simulink model "sopc_edge_detector"  (Simulink 6.3)
settings: Solver=FixedStepDiscrete  SolverMode=SingleTasking  StartTime=0.0  StopTime=307201.0  RelTol=1e-3
InitFcn:
  | ed_in_script
  | %% DSPBuilder Start
  | alt_dspbuilder_update_model(bdroot)
  | %% DSPBuilder End
StopFcn:
  | ed_out_script
libraries: allblocks_alteradspbuilder2 x63
settings Model: Creator=sichou  LastModifiedBy=LKONG
settings DataIOCC: SignalLoggingName=sigsOut
settings OptimizationCC: InlineInvariantSignals=on
settings DebuggingCC: AlgebraicLoopMsg=none  ArtificialAlgebraicLoopMsg=none  CheckExecutionContextPreStartOutputMsg=on  CheckExecutionContextRuntimeOutputMsg=on  SolverPrmCheckMsg=none
settings HardwareCC: TargetHWDeviceType=32-bit Generic  ProdEqTarget=off

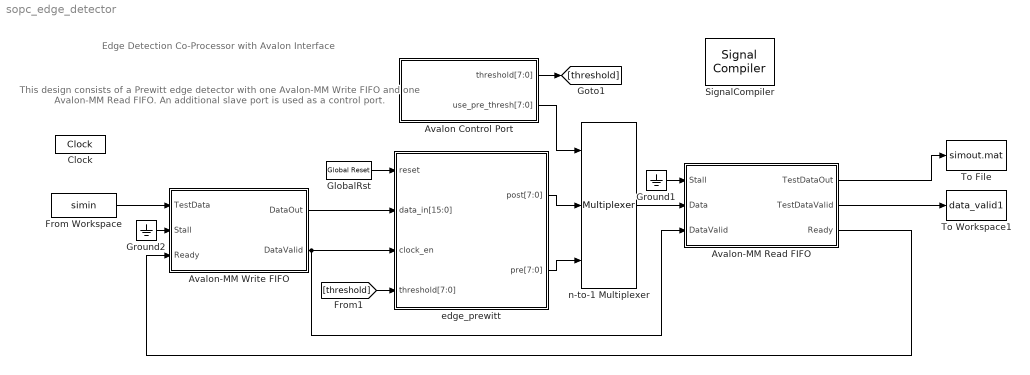
== system sopc_edge_detector ==
  note: Edge Detection Co-Processor
      | with Avalon Interface
  note: This design consists of a Prewitt edge detector with one Avalon-MM
      | Write FIFO and one Avalon-MM Read FIFO.  An additional slave port
      | is used as a control port.
  Avalon Control Port : Subsystem
      mask Type: SubSystem AlteraBlockSet
  Avalon-MM Read FIFO : Subsystem  mask(Avalon-MM Read FIFO AlteraBlockSet){sgn=Unsigned Integer, bwl=8, bwr=0, depth=16, burst=8}
      mask prompts: sgn "Data Type"; bwl "[number of bits].[]"; bwr "[].[number of bits]"; depth "FIFO Depth"; burst "Max Burst"
      mask help:
      | Avalon-MM Read FIFO
      |
      | Implements a FIFO with Avalon-MM connectivity. Accessed by other Avalon-MM peripherals to obtain datawhen connected in SOPC Builder.
      |
      | Inputs:
      | Stall - Connect to Simulink blocks.
      | 	Used to simulate stall conditions of the Avalon-MM bus.
      | Data - Connect to DSP Builder blocks.
      | 	Used to collect outgoing data from the user design.
      | DataValid - Connect to DSP Builder blocks.
      | 	Should be asserted whenever the signal on the Data port corresponds to real data.
      |
      | Outputs:
      | TestDataOut - Connect to Simulink blocks.
      | 	Corresponds to the data received over the Avalon-MM bus.
      | TestDataValid - Connect to Simulink blocks.
      | 	Asserted whenever TestDataOut corresponds to real data.
      | Ready	- Connect to DSP Builder blocks.
      | 	Used to indicate that the block is ready to receive data.
      mask init:
      | alt_dspbuilder_internal_AvalonFIFO_Init(gcb,1,1, bwl,bwr,depth,burst);
      settings: CopyFcn=set_param(gcbh,'LinkStatus','none');
      mask Help: helpview(fullfile(alt_dspbuilder_get_quartus_rootdir, 'dsp_builder', 'docs', 'AvalonReadFIFO.html'))
      mask StyleString: popup(Signed Integer|Signed Fractional|Unsigned Integer),edit,edit,edit,edit
      mask CallbackString: alt_dspbuilder_internal_AvalonFIFO_Init(gcb,1,0);||||
  Avalon-MM Write FIFO : Subsystem  mask(Avalon-MM Write FIFO AlteraBlockSet){sgn=Unsigned Integer, bwl=8, bwr=0, depth=16, burst=8}
      mask prompts: sgn "Data Type"; bwl "[number of bits].[]"; bwr "[].[number of bits]"; depth "FIFO Depth"; burst "Maximum Burst Size"
      mask help:
      | Avalon-MM Write FIFO
      |
      | Implements a FIFO with Avalon-MM connectivity. Used to receive data from other Avalon-MM peripheralswhen connected in SOPC Builder.
      |
      | Inputs:
      | TestData - Connect to Simulink blocks.
      | 	Used to provide simulation data to the Avalon-MM Write FIFO.
      | Stall - Connect to Simulink blocks.
      | 	Used to simulate stall conditions of the Avalon-MM bus.
      | Ready - Connect to DSP Builder blocks.
      | 	Used to indicate that the downstream hardware is ready for data.
      |
      | Outputs:
      | DataOut - Connect to DSP Builder blocks.
      | 	Corresponds to the oldest unsent data sample received on the TestData port.
      | DataValid - Connect to DSP Builder blocks.
      | 	Asserted whenever DataOut corresponds to real data.
      mask init:
      | alt_dspbuilder_internal_AvalonFIFO_Init(gcb,0,1, bwl,bwr,depth,burst);
      settings: CopyFcn=set_param(gcbh,'LinkStatus','none');
      mask Help: helpview(fullfile(alt_dspbuilder_get_quartus_rootdir, 'dsp_builder', 'docs', 'AvalonWriteFifo.html'))
      mask StyleString: popup(Signed Integer|Signed Fractional|Unsigned Integer),edit,edit,edit,edit
      mask CallbackString: alt_dspbuilder_internal_AvalonFIFO_Init(gcb,0,0);||||
  Clock : allblocks_alteradspbuilder2/Clock  ClockPeriod=100  ClockPeriodUnit=ns  SampleTime=1  SimulationStartCycle=5  PhaseOffset=0  Reset=aclr  ResetType=Active Low  Export=off
  From Workspace : FromWorkspace  VariableName=simin  SampleTime=1
  GlobalRst : allblocks_alteradspbuilder2/Global Reset  SpecifyClock=off
  Ground1 : Ground
  Ground2 : Ground
  SignalCompiler : allblocks_alteradspbuilder2/Signal Compiler  DeviceFamily=Stratix III  DeviceName=AUTO  EnableSignalTap=off  SignalTapDepth=128  UseBoardBlock=off  StpUseDefaultClock=on  StpClock=Clock
  To File : ToFile  Filename=simout.mat  MatrixName=simout
  To Workspace1 : ToWorkspace  VariableName=data_valid1  SampleTime=-1  SaveFormat=Array
  edge_prewitt : Subsystem
      mask Type: SubSystem AlteraBlockSet
  n-to-1 Multiplexer : allblocks_alteradspbuilder2/Multiplexer  numInputs=2  pipeline=0  oneHot=off  use_ena=off  use_aclr=off
  wires:
  Avalon-MM Write FIFO/1(DataOut) -> edge_prewitt/2(data_in[15:0])
  Avalon-MM Write FIFO/2(DataValid) -> edge_prewitt/3(clock_en), Avalon-MM Read FIFO/3(DataValid)
  Avalon-MM Read FIFO/3(Ready) -> Avalon-MM Write FIFO/3(Ready)
  GlobalRst/1 -> edge_prewitt/1(reset)
  Ground2/1 -> Avalon-MM Write FIFO/2(Stall)
  From Workspace/1 -> Avalon-MM Write FIFO/1(TestData)
  edge_prewitt/1(post[7:0]) -> n-to-1 Multiplexer/2
  Ground1/1 -> Avalon-MM Read FIFO/1(Stall)
  Avalon-MM Read FIFO/1(TestDataOut) -> To File/1
  Avalon-MM Read FIFO/2(TestDataValid) -> To Workspace1/1
  Avalon Control Port/2(use_pre_thresh[7:0]) -> n-to-1 Multiplexer/1
  n-to-1 Multiplexer/1 -> Avalon-MM Read FIFO/2(Data)
  edge_prewitt/2(pre[7:0]) -> n-to-1 Multiplexer/3
  Avalon Control Port/1(threshold[7:0]) -> [threshold]
  [threshold] -> edge_prewitt/4(threshold[7:0])

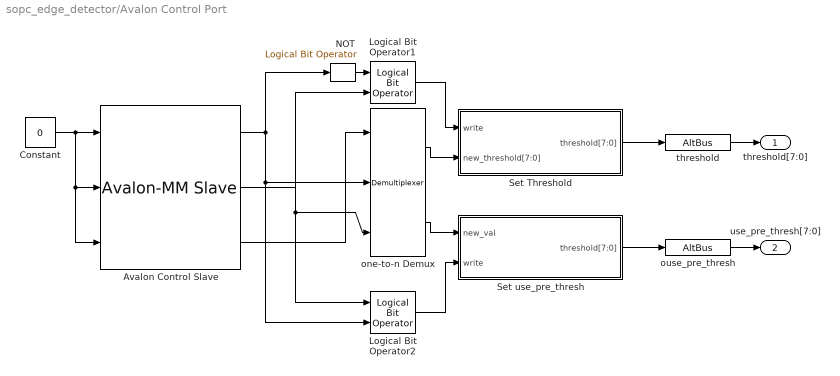
== system sopc_edge_detector/Avalon Control Port ==
  Avalon Control Slave : allblocks_alteradspbuilder2/Avalon-MM Slave  iofile=d:\wsTrunk\workspace\Documentation\DesignExamples\Tutorials\SOPCBuilder\AvalonFIFO\tb_sopc_edge_detector\sopc_edge_detector_Avalon+Control+Port_Avalon+Control+Slave_address.salt,d:\wsTrunk\workspace\Documentation\DesignExamples\Tutorials\SOPCBuilder\AvalonFIFO\tb_sopc_edge_detector\sopc_edge_detector_Avalon+Control+Port_Avalon+Control+Slave_write.salt,d:\wsTrunk\workspace\Documentation\DesignExamples\Tutorials\SOPCBuilder\AvalonFIFO\tb_sopc_edge_detector\sopc_edge_detector_Avalon+Control+Port_Avalon+Control+Slave_writedata.salt,  SpecifyClock=off  clock=clock  addrWidth=1  addrAlignment=Dynamic  addrType=Write  BusType=Unsigned Integer  bwl=8  bwr=0  byteEnable=off  flowCtrl=off  pipeline=off  waitStateFormat=Fixed  readWaitStateCycles=1  writeWaitStateCycles=0  readLatencyFormat=Fixed  readLatencyCycles=0  burst=off  maxBurst=8  irq=off  receiveBeginTransfer=off  useChipSelect=off  PORTTYPE=Output
  Constant : Constant  Value=0
  Logical Bit Operator1 : allblocks_alteradspbuilder2/Logical Bit Operator  LogicalOperator=AND  user_inputs=2
  Logical Bit Operator2 : allblocks_alteradspbuilder2/Logical Bit Operator  LogicalOperator=AND  user_inputs=2
  NOT : allblocks_alteradspbuilder2/Logical Bit Operator  LogicalOperator=NOT  user_inputs=2
  Set Threshold : Subsystem
      mask Type: SubSystem AlteraBlockSet
  Set use_pre_thresh : Subsystem
      mask Type: SubSystem AlteraBlockSet
  one-to-n Demux : allblocks_alteradspbuilder2/Demultiplexer  numOutputs=2  use_ena=on  use_sclr=off
  ouse_pre_thresh : allblocks_alteradspbuilder2/AltBus  BusType=Signed Integer  bwl=8  bwr=0  saturate=off
  threshold : allblocks_alteradspbuilder2/AltBus  BusType=Signed Integer  bwl=8  bwr=0  saturate=off
  threshold[7:0] : Outport
  use_pre_thresh[7:0] : Outport  Port=2
  wires:
  ouse_pre_thresh/1 -> use_pre_thresh[7:0]/1
  Avalon Control Slave/1 -> one-to-n Demux/2, Logical Bit Operator2/2, NOT/1
  Avalon Control Slave/2 -> Logical Bit Operator1/2, one-to-n Demux/3, Logical Bit Operator2/1
  Avalon Control Slave/3 -> one-to-n Demux/1
  one-to-n Demux/1 -> Set Threshold/2(new_threshold[7:0])
  Set use_pre_thresh/1(threshold[7:0]) -> ouse_pre_thresh/1
  NOT/1 -> Logical Bit Operator1/1
  Logical Bit Operator1/1 -> Set Threshold/1(write)
  Logical Bit Operator2/1 -> Set use_pre_thresh/2(write)
  one-to-n Demux/2 -> Set use_pre_thresh/1(new_val)
  threshold/1 -> threshold[7:0]/1
  Set Threshold/1(threshold[7:0]) -> threshold/1
  Constant/1 -> Avalon Control Slave/1, Avalon Control Slave/2, Avalon Control Slave/3

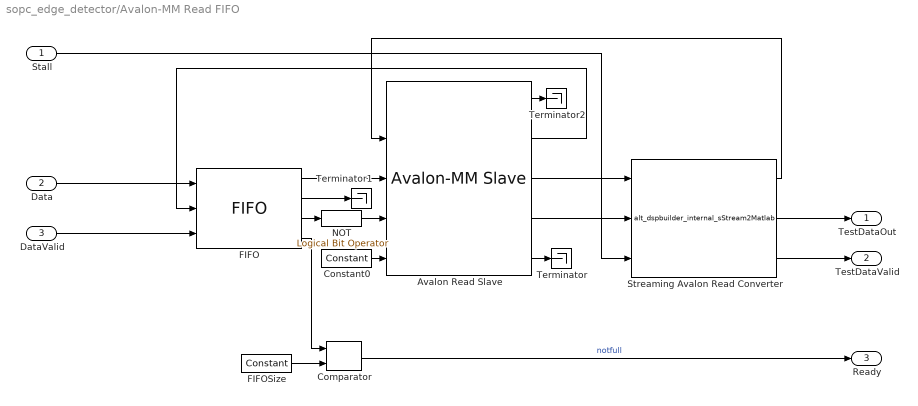
== system sopc_edge_detector/Avalon-MM Read FIFO ==
  Stall : Inport
  Data : Inport  Port=2
  DataValid : Inport  Port=3
  Avalon Read Slave : allblocks_alteradspbuilder2/Avalon-MM Slave  iofile=d:\wsTrunk\workspace\Documentation\DesignExamples\Tutorials\SOPCBuilder\AvalonFIFO\tb_sopc_edge_detector\sopc_edge_detector_Avalon-MM+Read+FIFO_Avalon+Read+Slave_address.salt,d:\wsTrunk\workspace\Documentation\DesignExamples\Tutorials\SOPCBuilder\AvalonFIFO\tb_sopc_edge_detector\sopc_edge_detector_Avalon-MM+Read+FIFO_Avalon+Read+Slave_read.salt,d:\wsTrunk\workspace\Documentation\DesignExamples\Tutorials\SOPCBuilder\AvalonFIFO\tb_sopc_edge_detector\sopc_edge_detector_Avalon-MM+Read+FIFO_Avalon+Read+Slave_readdata.capture,d:\wsTrunk\workspace\Documentation\DesignExamples\Tutorials\SOPCBuilder\AvalonFIFO\tb_sopc_edge_detector\sopc_edge_detector_Avalon-MM+Read+FIFO_Avalon+Read+Slave_dataavailable.capture,d:\wsTrunk\workspace\Documentation\DesignExamples\Tutorials\SOPCBuilder\AvalonFIFO\tb_sopc_edge_detector\sopc_edge_detector_Avalon-MM+Read+FIFO_Avalon+Read+Slave_endofpacket.capture,  SpecifyClock=off  clock=clock  addrWidth=2  addrAlignment=Dynamic  addrType=Read  BusType=Unsigned Integer  bwl=bwl  bwr=bwr  byteEnable=off  flowCtrl=on  pipeline=off  waitStateFormat=Fixed  readWaitStateCycles=0  writeWaitStateCycles=0  readLatencyFormat=Fixed  readLatencyCycles=0  burst=off  maxBurst=burst  irq=off  receiveBeginTransfer=off  useChipSelect=off  PORTTYPE=Output
  Comparator : allblocks_alteradspbuilder2/Comparator  direction=a < b
  Constant0 : allblocks_alteradspbuilder2/Constant  mask_cst=0  BusType=Single Bit  bwl=1  bwr=0  SpecifyClock=off
  FIFO : allblocks_alteradspbuilder2/FIFO  numwords=depth  BusType=Unsigned Integer  bwl=bwl  bwr=bwr  ram_type=AUTO  use_sclr=off  use_les_only=off  showahead_mode=off
  FIFOSize : allblocks_alteradspbuilder2/Constant  mask_cst=depth - 2  BusType=Unsigned Integer  bwl=ceil(log2(depth -1))  bwr=0  SpecifyClock=off
  NOT : allblocks_alteradspbuilder2/Logical Bit Operator  LogicalOperator=NOT  user_inputs=2
  Streaming Avalon Read Converter : S-Function  FunctionName=alt_dspbuilder_internal_sStream2Matlab  Parameters=-1
      mask Display:
      | port_label('input', 1, 'ReadData');
      | port_label('input', 2, 'DataAvailable');
      | port_label('input', 3, 'Stall');
      | port_label('output', 1, 'Read');
      | port_label('output', 2, 'TestData');
      | port_label('output', 3, 'TestDataValid');
  Terminator : Terminator
  Terminator1 : Terminator
  Terminator2 : Terminator
  TestDataOut : Outport
  TestDataValid : Outport  Port=2
  Ready : Outport  Port=3
  wires:
  DataValid/1 -> FIFO/3
  FIFO/3 -> NOT/1
  NOT/1 -> Avalon Read Slave/4
  Data/1 -> FIFO/1
  FIFO/1 -> Avalon Read Slave/3
  Avalon Read Slave/2 -> FIFO/2
  Streaming Avalon Read Converter/2 -> TestDataOut/1
  Streaming Avalon Read Converter/3 -> TestDataValid/1
  Streaming Avalon Read Converter/1 -> Avalon Read Slave/2
  Avalon Read Slave/3 -> Streaming Avalon Read Converter/1
  Constant0/1 -> Avalon Read Slave/5
  FIFO/4 -> Comparator/1
  Comparator/1 -> Ready/1  "notfull"
  Stall/1 -> Streaming Avalon Read Converter/3
  Avalon Read Slave/4 -> Streaming Avalon Read Converter/2
  Avalon Read Slave/5 -> Terminator/1
  FIFOSize/1 -> Comparator/2
  FIFO/2 -> Terminator1/1
  Avalon Read Slave/1 -> Terminator2/1

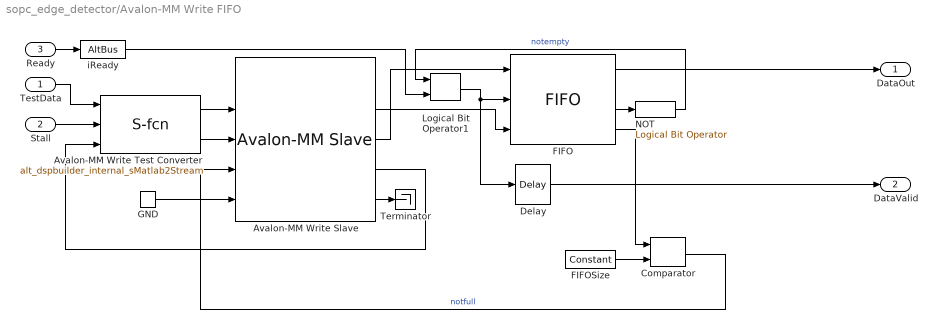
== system sopc_edge_detector/Avalon-MM Write FIFO ==
  TestData : Inport
  Stall : Inport  Port=2
  Ready : Inport  Port=3
  Avalon-MM Write Slave : allblocks_alteradspbuilder2/Avalon-MM Slave  iofile=d:\wsTrunk\workspace\Documentation\DesignExamples\Tutorials\SOPCBuilder\AvalonFIFO\tb_sopc_edge_detector\sopc_edge_detector_Avalon-MM+Write+FIFO_Avalon-MM+Write+Slave_address.salt,d:\wsTrunk\workspace\Documentation\DesignExamples\Tutorials\SOPCBuilder\AvalonFIFO\tb_sopc_edge_detector\sopc_edge_detector_Avalon-MM+Write+FIFO_Avalon-MM+Write+Slave_write.salt,d:\wsTrunk\workspace\Documentation\DesignExamples\Tutorials\SOPCBuilder\AvalonFIFO\tb_sopc_edge_detector\sopc_edge_detector_Avalon-MM+Write+FIFO_Avalon-MM+Write+Slave_writedata.salt,d:\wsTrunk\workspace\Documentation\DesignExamples\Tutorials\SOPCBuilder\AvalonFIFO\tb_sopc_edge_detector\sopc_edge_detector_Avalon-MM+Write+FIFO_Avalon-MM+Write+Slave_readyfordata.capture,d:\wsTrunk\workspace\Documentation\DesignExamples\Tutorials\SOPCBuilder\AvalonFIFO\tb_sopc_edge_detector\sopc_edge_detector_Avalon-MM+Write+FIFO_Avalon-MM+Write+Slave_endofpacket.capture,  SpecifyClock=off  clock=clock  addrWidth=2  addrAlignment=Dynamic  addrType=Write  BusType=Unsigned Integer  bwl=bwl  bwr=bwr  byteEnable=off  flowCtrl=on  pipeline=off  waitStateFormat=Fixed  readWaitStateCycles=0  writeWaitStateCycles=0  readLatencyFormat=Fixed  readLatencyCycles=0  burst=off  maxBurst=burst  irq=off  receiveBeginTransfer=off  useChipSelect=off  PORTTYPE=Output
  Avalon-MM Write Test Converter : S-Function  FunctionName=alt_dspbuilder_internal_sMatlab2Stream  Parameters=-1 1000000
      mask Display:
      | port_label('input', 1, 'TestData');
      | port_label('input', 2, 'Stall');
      | port_label('input', 3, 'Ready');
      | port_label('output', 1, 'Write');
      | port_label('output', 2, 'WriteData');
  Comparator : allblocks_alteradspbuilder2/Comparator  direction=a < b
  Delay : allblocks_alteradspbuilder2/Delay  pipeline=1  ClockPhase=1  use_ena=off  use_sclr=off  use_init=off  reset_value=1
  FIFO : allblocks_alteradspbuilder2/FIFO  numwords=depth  BusType=Unsigned Integer  bwl=bwl  bwr=bwr  ram_type=AUTO  use_sclr=off  use_les_only=off  showahead_mode=off
  FIFOSize : allblocks_alteradspbuilder2/Constant  mask_cst=depth -2  BusType=Unsigned Integer  bwl=ceil(log2(depth-1))  bwr=0  SpecifyClock=off
  GND : allblocks_alteradspbuilder2/GND  SpecifyClock=off
  Logical Bit Operator1 : allblocks_alteradspbuilder2/Logical Bit Operator  LogicalOperator=AND  user_inputs=2
  NOT : allblocks_alteradspbuilder2/Logical Bit Operator  LogicalOperator=NOT  user_inputs=2
  Terminator : Terminator
  iReady : allblocks_alteradspbuilder2/AltBus  BusType=Single Bit  bwl=1  bwr=0  saturate=off
  DataOut : Outport
  DataValid : Outport  Port=2
  wires:
  Ready/1 -> iReady/1
  Avalon-MM Write Slave/3 -> FIFO/1
  Avalon-MM Write Slave/2 -> FIFO/3
  FIFO/3 -> NOT/1
  FIFO/1 -> DataOut/1
  Avalon-MM Write Test Converter/1 -> Avalon-MM Write Slave/2
  Avalon-MM Write Slave/4 -> Avalon-MM Write Test Converter/3
  TestData/1 -> Avalon-MM Write Test Converter/1
  GND/1 -> Avalon-MM Write Slave/5
  NOT/1 -> Logical Bit Operator1/1  "notempty"
  iReady/1 -> Logical Bit Operator1/2
  Delay/1 -> DataValid/1
  Avalon-MM Write Test Converter/2 -> Avalon-MM Write Slave/3
  Stall/1 -> Avalon-MM Write Test Converter/2
  Avalon-MM Write Slave/5 -> Terminator/1
  Comparator/1 -> Avalon-MM Write Slave/4  "notfull"
  FIFOSize/1 -> Comparator/2
  FIFO/4 -> Comparator/1
  Logical Bit Operator1/1 -> FIFO/2, Delay/1

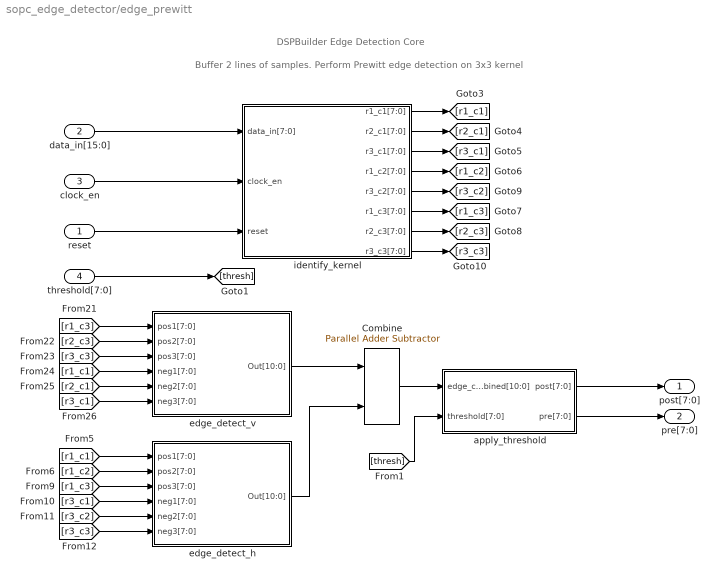
== system sopc_edge_detector/edge_prewitt ==
  note: Buffer 2 lines of samples.
      | Perform Prewitt edge detection on 3x3 kernel
  note: DSPBuilder Edge Detection Core
  reset : Inport
  data_in[15:0] : Inport  Port=2
  clock_en : Inport  Port=3
  threshold[7:0] : Inport  Port=4
  Combine : allblocks_alteradspbuilder2/Parallel Adder Subtractor  number_of_inputs=2  direction=+  use_pipeline=off  phase_selection=1  use_ena=off  use_aclr=off
  apply_threshold : Subsystem
      mask Type: SubSystem AlteraBlockSet
  edge_detect_h : Subsystem  AncestorBlock=ALTELINK/AltLab/HDL SubSystem
      mask Type: SubSystem AlteraBlockSet
  edge_detect_v : Subsystem  AncestorBlock=ALTELINK/AltLab/HDL SubSystem
      mask Type: SubSystem AlteraBlockSet
  identify_kernel : Subsystem
      mask Type: SubSystem AlteraBlockSet
  post[7:0] : Outport
  pre[7:0] : Outport  Port=2
  wires:
  clock_en/1 -> identify_kernel/2(clock_en)
  data_in[15:0]/1 -> identify_kernel/1(data_in[7:0])
  reset/1 -> identify_kernel/3(reset)
  apply_threshold/1(post[7:0]) -> post[7:0]/1
  identify_kernel/8(r3_c3[7:0]) -> [r3_c3]
  identify_kernel/5(r3_c2[7:0]) -> [r3_c2]
  identify_kernel/7(r2_c3[7:0]) -> [r2_c3]
  identify_kernel/6(r1_c3[7:0]) -> [r1_c3]
  identify_kernel/4(r1_c2[7:0]) -> [r1_c2]
  identify_kernel/3(r3_c1[7:0]) -> [r3_c1]
  identify_kernel/2(r2_c1[7:0]) -> [r2_c1]
  identify_kernel/1(r1_c1[7:0]) -> [r1_c1]
  [r3_c1] -> edge_detect_v/6(neg3[7:0])
  [r2_c1] -> edge_detect_v/5(neg2[7:0])
  [r1_c1] -> edge_detect_v/4(neg1[7:0])
  [r3_c3] -> edge_detect_v/3(pos3[7:0])
  [r2_c3] -> edge_detect_v/2(pos2[7:0])
  [r1_c3] -> edge_detect_v/1(pos1[7:0])
  apply_threshold/2(pre[7:0]) -> pre[7:0]/1
  [r3_c3] -> edge_detect_h/6(neg3[7:0])
  [r3_c2] -> edge_detect_h/5(neg2[7:0])
  [r3_c1] -> edge_detect_h/4(neg1[7:0])
  [r1_c3] -> edge_detect_h/3(pos3[7:0])
  [r1_c2] -> edge_detect_h/2(pos2[7:0])
  [r1_c1] -> edge_detect_h/1(pos1[7:0])
  Combine/1 -> apply_threshold/1(edge_combined[10:0])
  edge_detect_v/1(Out[10:0]) -> Combine/1
  edge_detect_h/1(Out[10:0]) -> Combine/2
  threshold[7:0]/1 -> [thresh]
  [thresh] -> apply_threshold/2(threshold[7:0])

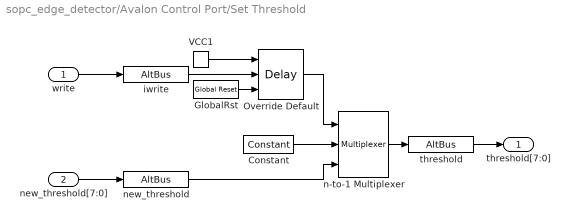
== system sopc_edge_detector/Avalon Control Port/Set Threshold ==
  write : Inport
  new_threshold[7:0] : Inport  Port=2
  Constant : allblocks_alteradspbuilder2/Constant  mask_cst=50  BusType=Unsigned Integer  bwl=8  bwr=0  SpecifyClock=off
  GlobalRst : allblocks_alteradspbuilder2/Global Reset  SpecifyClock=off
  Override Default : allblocks_alteradspbuilder2/Delay  pipeline=1  ClockPhase=1  use_ena=on  use_sclr=on  use_init=off  reset_value=1
  VCC1 : allblocks_alteradspbuilder2/VCC  SpecifyClock=off
  iwrite : allblocks_alteradspbuilder2/AltBus  BusType=Single Bit  bwl=1  bwr=0  saturate=off
  n-to-1 Multiplexer : allblocks_alteradspbuilder2/Multiplexer  numInputs=2  pipeline=0  oneHot=off  use_ena=off  use_aclr=off
  new_threshold : allblocks_alteradspbuilder2/AltBus  BusType=Unsigned Integer  bwl=8  bwr=0  saturate=off
  threshold : allblocks_alteradspbuilder2/AltBus  BusType=Signed Integer  bwl=8  bwr=0  saturate=off
  threshold[7:0] : Outport
  wires:
  threshold/1 -> threshold[7:0]/1
  new_threshold[7:0]/1 -> new_threshold/1
  write/1 -> iwrite/1
  Override Default/1 -> n-to-1 Multiplexer/1
  new_threshold/1 -> n-to-1 Multiplexer/3
  n-to-1 Multiplexer/1 -> threshold/1
  VCC1/1 -> Override Default/1
  iwrite/1 -> Override Default/2
  GlobalRst/1 -> Override Default/3
  Constant/1 -> n-to-1 Multiplexer/2

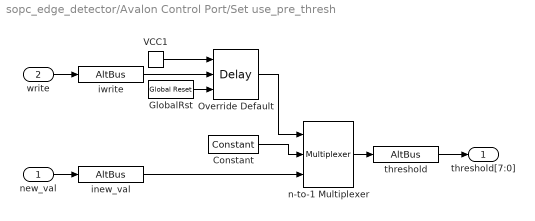
== system sopc_edge_detector/Avalon Control Port/Set use_pre_thresh ==
  new_val : Inport
  write : Inport  Port=2
  Constant : allblocks_alteradspbuilder2/Constant  mask_cst=0  BusType=Unsigned Integer  bwl=1  bwr=0  SpecifyClock=off
  GlobalRst : allblocks_alteradspbuilder2/Global Reset  SpecifyClock=off
  Override Default : allblocks_alteradspbuilder2/Delay  pipeline=1  ClockPhase=1  use_ena=on  use_sclr=on  use_init=off  reset_value=1
  VCC1 : allblocks_alteradspbuilder2/VCC  SpecifyClock=off
  inew_val : allblocks_alteradspbuilder2/AltBus  BusType=Single Bit  bwl=1  bwr=0  saturate=off
  iwrite : allblocks_alteradspbuilder2/AltBus  BusType=Single Bit  bwl=1  bwr=0  saturate=off
  n-to-1 Multiplexer : allblocks_alteradspbuilder2/Multiplexer  numInputs=2  pipeline=0  oneHot=off  use_ena=off  use_aclr=off
  threshold : allblocks_alteradspbuilder2/AltBus  BusType=Signed Integer  bwl=8  bwr=0  saturate=off
  threshold[7:0] : Outport
  wires:
  GlobalRst/1 -> Override Default/3
  iwrite/1 -> Override Default/2
  VCC1/1 -> Override Default/1
  n-to-1 Multiplexer/1 -> threshold/1
  inew_val/1 -> n-to-1 Multiplexer/3
  Override Default/1 -> n-to-1 Multiplexer/1
  write/1 -> iwrite/1
  new_val/1 -> inew_val/1
  threshold/1 -> threshold[7:0]/1
  Constant/1 -> n-to-1 Multiplexer/2

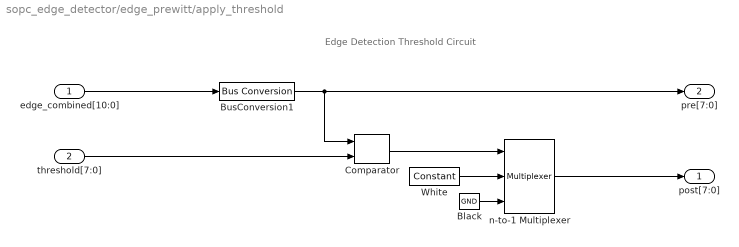
== system sopc_edge_detector/edge_prewitt/apply_threshold ==
  note: Edge Detection Threshold Circuit
  edge_combined[10:0] : Inport
  threshold[7:0] : Inport  Port=2
  Black : allblocks_alteradspbuilder2/GND  SpecifyClock=off
  BusConversion1 : allblocks_alteradspbuilder2/Bus Conversion  BusType=Unsigned Integer  ibwl=11  ibwr=0  bwl=8  bwr=0  bitToConnectToOutputLSB=0  round=off  saturate=on
  Comparator : allblocks_alteradspbuilder2/Comparator  direction=a < b
  White : allblocks_alteradspbuilder2/Constant  mask_cst=255  BusType=Unsigned Integer  bwl=8  bwr=0  SpecifyClock=off
  n-to-1 Multiplexer : allblocks_alteradspbuilder2/Multiplexer  numInputs=2  pipeline=0  oneHot=off  use_ena=off  use_aclr=off
  post[7:0] : Outport
  pre[7:0] : Outport  Port=2
  wires:
  Black/1 -> n-to-1 Multiplexer/3
  White/1 -> n-to-1 Multiplexer/2
  n-to-1 Multiplexer/1 -> post[7:0]/1
  edge_combined[10:0]/1 -> BusConversion1/1
  BusConversion1/1 -> Comparator/1, pre[7:0]/1
  Comparator/1 -> n-to-1 Multiplexer/1
  threshold[7:0]/1 -> Comparator/2

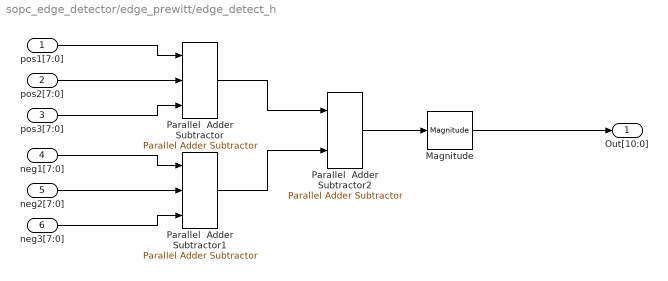
== system sopc_edge_detector/edge_prewitt/edge_detect_h ==
  pos1[7:0] : Inport
  pos2[7:0] : Inport  Port=2
  pos3[7:0] : Inport  Port=3
  neg1[7:0] : Inport  Port=4
  neg2[7:0] : Inport  Port=5
  neg3[7:0] : Inport  Port=6
  Magnitude : allblocks_alteradspbuilder2/Magnitude
  Parallel  Adder Subtractor : allblocks_alteradspbuilder2/Parallel Adder Subtractor  number_of_inputs=3  direction=+  use_pipeline=off  phase_selection=1  use_ena=off  use_aclr=off
  Parallel  Adder Subtractor1 : allblocks_alteradspbuilder2/Parallel Adder Subtractor  number_of_inputs=3  direction=+  use_pipeline=off  phase_selection=1  use_ena=off  use_aclr=off
  Parallel  Adder Subtractor2 : allblocks_alteradspbuilder2/Parallel Adder Subtractor  number_of_inputs=2  direction=+-  use_pipeline=off  phase_selection=1  use_ena=off  use_aclr=off
  Out[10:0] : Outport
  wires:
  Parallel  Adder Subtractor2/1 -> Magnitude/1
  Parallel  Adder Subtractor/1 -> Parallel  Adder Subtractor2/1
  Parallel  Adder Subtractor1/1 -> Parallel  Adder Subtractor2/2
  pos1[7:0]/1 -> Parallel  Adder Subtractor/1
  pos2[7:0]/1 -> Parallel  Adder Subtractor/2
  pos3[7:0]/1 -> Parallel  Adder Subtractor/3
  neg1[7:0]/1 -> Parallel  Adder Subtractor1/1
  neg2[7:0]/1 -> Parallel  Adder Subtractor1/2
  neg3[7:0]/1 -> Parallel  Adder Subtractor1/3
  Magnitude/1 -> Out[10:0]/1

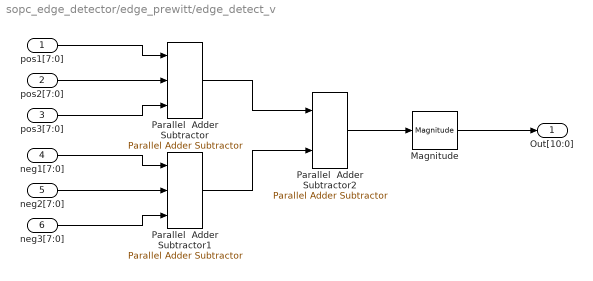
== system sopc_edge_detector/edge_prewitt/edge_detect_v ==
  pos1[7:0] : Inport
  pos2[7:0] : Inport  Port=2
  pos3[7:0] : Inport  Port=3
  neg1[7:0] : Inport  Port=4
  neg2[7:0] : Inport  Port=5
  neg3[7:0] : Inport  Port=6
  Magnitude : allblocks_alteradspbuilder2/Magnitude
  Parallel  Adder Subtractor : allblocks_alteradspbuilder2/Parallel Adder Subtractor  number_of_inputs=3  direction=+  use_pipeline=off  phase_selection=1  use_ena=off  use_aclr=off
  Parallel  Adder Subtractor1 : allblocks_alteradspbuilder2/Parallel Adder Subtractor  number_of_inputs=3  direction=+  use_pipeline=off  phase_selection=1  use_ena=off  use_aclr=off
  Parallel  Adder Subtractor2 : allblocks_alteradspbuilder2/Parallel Adder Subtractor  number_of_inputs=2  direction=+-  use_pipeline=off  phase_selection=1  use_ena=off  use_aclr=off
  Out[10:0] : Outport
  wires:
  Magnitude/1 -> Out[10:0]/1
  neg3[7:0]/1 -> Parallel  Adder Subtractor1/3
  neg2[7:0]/1 -> Parallel  Adder Subtractor1/2
  neg1[7:0]/1 -> Parallel  Adder Subtractor1/1
  pos3[7:0]/1 -> Parallel  Adder Subtractor/3
  pos2[7:0]/1 -> Parallel  Adder Subtractor/2
  pos1[7:0]/1 -> Parallel  Adder Subtractor/1
  Parallel  Adder Subtractor1/1 -> Parallel  Adder Subtractor2/2
  Parallel  Adder Subtractor/1 -> Parallel  Adder Subtractor2/1
  Parallel  Adder Subtractor2/1 -> Magnitude/1

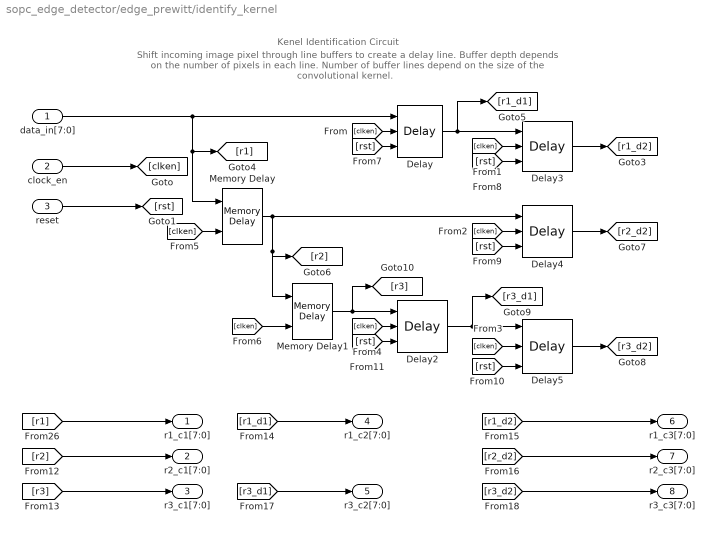
== system sopc_edge_detector/edge_prewitt/identify_kernel ==
  note: Kenel Identification Circuit
  note: Shift incoming image pixel through line buffers to create a delay line.  Buffer depth depends on the number of pixels
      | in each line.  Number of buffer lines depend on the size of the convolutional kernel.
  data_in[7:0] : Inport
  clock_en : Inport  Port=2
  reset : Inport  Port=3
  Delay{,2..3,5} (4 alike) : allblocks_alteradspbuilder2/Delay  pipeline=1  ClockPhase=1  use_ena=on  use_sclr=on  use_init=off  reset_value=1
  Delay4 : allblocks_alteradspbuilder2/Delay  pipeline=2  ClockPhase=1  use_ena=on  use_sclr=on  use_init=off  reset_value=1
  Memory Delay : allblocks_alteradspbuilder2/Memory Delay  BusType=Inferred  bwl=8  bwr=0  pipeline=640  ram_type=AUTO  use_ena=on  use_sclr=off
  Memory Delay1 : allblocks_alteradspbuilder2/Memory Delay  BusType=Inferred  bwl=8  bwr=0  pipeline=640  ram_type=AUTO  use_ena=on  use_sclr=off
  r1_c1[7:0] : Outport
  r2_c1[7:0] : Outport  Port=2
  r3_c1[7:0] : Outport  Port=3
  r1_c2[7:0] : Outport  Port=4
  r3_c2[7:0] : Outport  Port=5
  r1_c3[7:0] : Outport  Port=6
  r2_c3[7:0] : Outport  Port=7
  r3_c3[7:0] : Outport  Port=8
  wires:
  [r3_d2] -> r3_c3[7:0]/1
  [r3_d1] -> r3_c2[7:0]/1
  [r2_d2] -> r2_c3[7:0]/1
  [r1_d2] -> r1_c3[7:0]/1
  [r1_d1] -> r1_c2[7:0]/1
  [r3] -> r3_c1[7:0]/1
  [r2] -> r2_c1[7:0]/1
  [r1] -> r1_c1[7:0]/1
  reset/1 -> [rst]
  clock_en/1 -> [clken]
  Delay5/1 -> [r3_d2]
  Delay4/1 -> [r2_d2]
  Delay3/1 -> [r1_d2]
  data_in[7:0]/1 -> Delay/1, Memory Delay/1, [r1]
  Delay2/1 -> [r3_d1], Delay5/1
  Delay/1 -> [r1_d1], Delay3/1
  [rst] -> Delay5/3
  [rst] -> Delay4/3
  [rst] -> Delay2/3
  [rst] -> Delay3/3
  [rst] -> Delay/3
  [clken] -> Memory Delay1/2
  [clken] -> Memory Delay/2
  [clken] -> Delay2/2
  [clken] -> Delay5/2
  [clken] -> Delay4/2
  [clken] -> Delay3/2
  [clken] -> Delay/2
  Memory Delay1/1 -> [r3], Delay2/1
  Memory Delay/1 -> [r2], Memory Delay1/1, Delay4/1
